simulink model "Subsystem"  (R2020b)
settings: Solver=VariableStepAuto  StartTime=0.0  StopTime=10.0  RelTol=1e-3
settings Model: Creator=shivanshu shukla  LastModifiedBy=shivanshu shukla
settings DataIOCC: SaveOutput=off  SaveTime=off

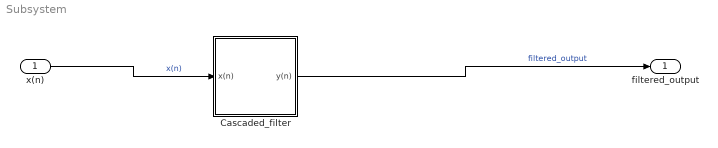
== system Subsystem ==
  x(n) : Inport  OutDataTypeStr=double  PortDimensions=1  SampleTime=[0,1]
  Cascaded_filter : Subsystem
  filtered_output : Outport  OutDataTypeStr=double  PortDimensions=1  SampleTime=[0,1]
  wires:
  Cascaded_filter/1(y(n)) -> filtered_output/1  "filtered_output"
  x(n)/1 -> Cascaded_filter/1(x(n))  "x(n)"

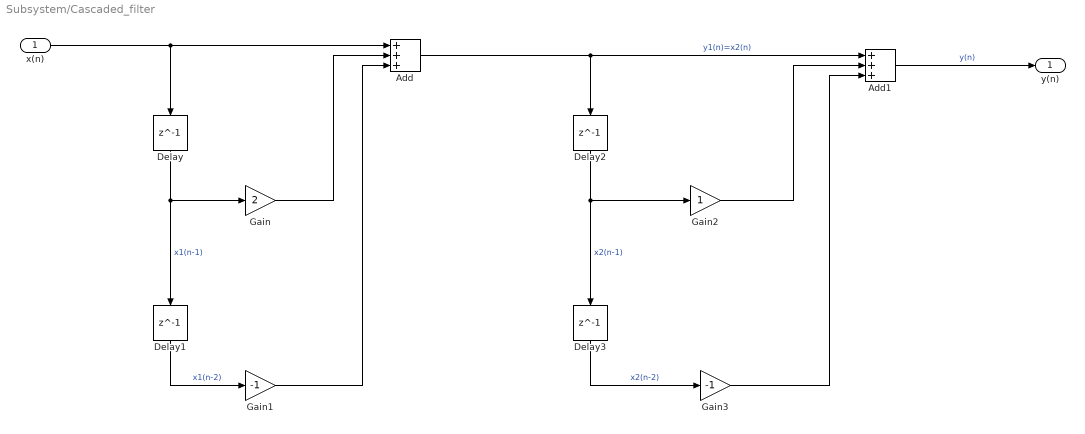
== system Subsystem/Cascaded_filter ==
  x(n) : Inport
  Add : Sum  Inputs=+++
  Add1 : Sum  Inputs=+++
  Delay{,1..3} (4 alike) : Delay  DelayLength=1
  Gain : Gain  Gain=2
  Gain1 : Gain  Gain=-1
  Gain2 : Gain
  Gain3 : Gain  Gain=-1
  y(n) : Outport
  wires:
  Gain1/1 -> Add/3
  Delay3/1 -> Gain3/1  "x2(n-2)"
  Gain/1 -> Add/2
  Delay2/1 -> Delay3/1, Gain2/1  "x2(n-1)"
  Gain2/1 -> Add1/2
  Delay1/1 -> Gain1/1  "x1(n-2)"
  Add1/1 -> y(n)/1  "y(n)"
  Gain3/1 -> Add1/3
  Delay/1 -> Gain/1, Delay1/1  "x1(n-1)"
  x(n)/1 -> Delay/1, Add/1
  Add/1 -> Delay2/1, Add1/1  "y1(n)=x2(n)"
